simulink subsystem "controller_skeleton_FILTERED"  (R2023b)
settings: Solver=FixedStepDiscrete  StartTime=0.0  StopTime=10.0  RelTol=1e-3  EnableMultiTasking=on
values from neighbouring files (symbols this model uses):
  tvs =     [tvs_parameters.mat]
settings Model: Creator=Inver  LastModifiedBy=Inver
settings SolverCC: AutoInsertRateTranBlk=on
settings DataIOCC: SaveOutput=off  SaveTime=off
settings OptimizationCC: DefaultParameterBehavior=Inlined  InlineInvariantSignals=on  EnhancedBackFolding=on  PassReuseOutputArgsAs=Individual arguments  StateBitsets=on  DataBitsets=on  ZeroExternalMemoryAtStartup=off  ZeroInternalMemoryAtStartup=off  NoFixptDivByZeroProtection=on  LifeSpan=1  OptimizeBlockOrder=speed  DifferentSizesBufferReuse=on  EfficientTunableParamExpr=on
settings DebuggingCC: ParameterTunabilityLossMsg=error
settings HardwareCC: ProdBitPerPointer=32  ProdBitPerSizeT=32  ProdBitPerPtrDiffT=32  ProdLargestAtomicFloat=None  ProdIntDivRoundTo=Floor  ProdWordSize=32  ProdHWDeviceType=Generic->Custom
settings SFSimCC: MATLABDynamicMemAlloc=off
settings RTWCC: Description=Embedded Coder  SystemTargetFile=ert.tlc  TLCOptions=-p0  GenCodeOnly=on  TemplateMakefile=ert_default_tmf  GenerateReport=on  RTWVerbose=off  IncludeHyperlinkInReport=on  LaunchReport=on
settings CodeAppCC: ForceParamTrailComments=on  IgnoreCustomStorageClasses=off  OperatorAnnotations=on  SimulinkDataObjDesc=on  SFDataObjDesc=on  CustomSymbolStrGlobalVar=rt$N$M  CustomSymbolStrType=$N$M  CustomSymbolStrFcn=$N$M$F  CustomSymbolStrMacro=$N$M  InsertBlockDesc=on
settings ERTTargetCC: TargetLangStandard=C99 (ISO)  CodeReplacementLibrary=ISO_C  GenerateSampleERTMain=on  IncludeMdlTerminateFcn=off  SuppressErrorStatus=on  SupportAbsoluteTime=off  PurelyIntegerCode=on  SupportNonFinite=off  SupportComplex=off  InlinedParameterPlacement=NonHierarchical  RootIOFormat=Structure reference  ERTCustomFileTemplate=example_file_process.tlc

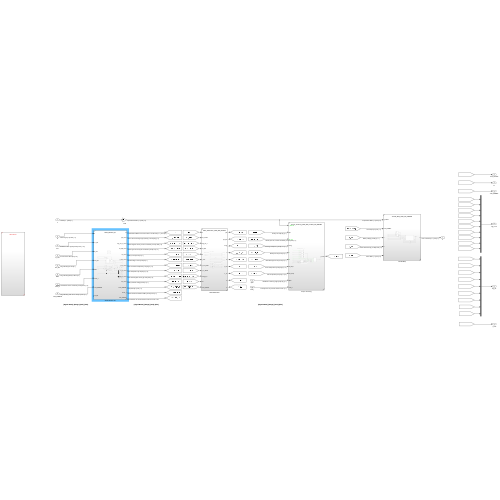
[thumbnail: Simulink's stored preview of the top-level diagram]
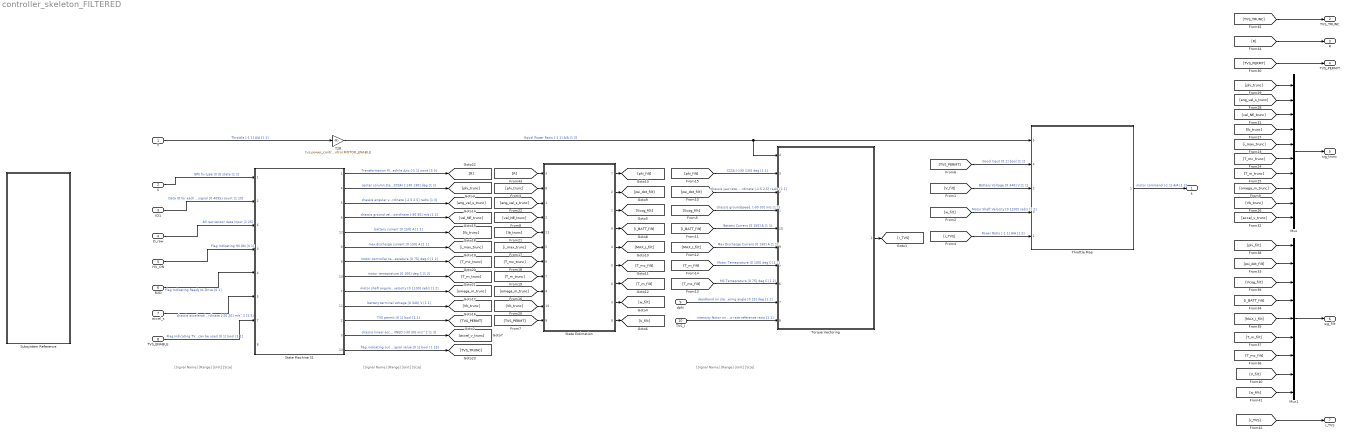
== system controller_skeleton_FILTERED ==
  note: [Signal Name] [Range] [Unit] [Size]
  note: [Signal Name] [Range] [Unit] [Size]
  note: [Signal Name] [Range] [Unit] [Size]
  T : Inport
  S : Inport  Port=2
  ID1 : Inport  Port=3
  D_raw : Inport  Port=4
  HV_ON : Inport  Port=5
  R2D : Inport  Port=6
  accel_s : Inport  Port=7
  TVS_ENABLE : Inport  Port=8
  dphi : Inport  Port=9
  TVS_I : Inport  Port=10
  Mux : Mux  Inputs=10
  Mux1 : Mux  Inputs=9
  State Estimation : Subsystem  ReferencedSubsystem=State_Estimation_2WD_NO_REGEN
      settings: PortSchema="{\"entries\":[{\"content\":{\"sides\":[{\"content\":{\"connectorIds\":[\"In3\",\"In8\",\"In1\",\"In2\",\"In11\",\"In5\",\"In6\",\"In7\",\"In4\",\"In10\",\"In9\"]},\"type\":\"ConnectorPlacement.EquallySpacedRectSide\",\"uuid\":\"a788c4af-c868-4742-81ae-137d8550b7dd\"},{\"content\":{\"connectorIds\":[\"Out7\",\"Out2\",\"Out1\",\"Out9\",\"Out4\",\"Out5\",\"Out6\",\"Out3\",\"Out8\"],\"side\":\"RIGHT\"},\"type\":\"ConnectorPlacement.EquallySpacedRectSide\",\"uuid\":\"40c1d3ed-7f96-4f50-8201-1fa73cbd293c\"},{\"content\":{\"side\":\"TOP\"},\"type\":\"ConnectorPlacement.EquallySpacedRectSide\",\"uuid\":\"412486a9-9897-40de-926c-efa6067c47b5\"}]},\"type\":\"ConnectorPlacement.EquallySpacedConnector\",\"uuid\":\"e2349428-ea4b-4d6c-9a0f-70e14711b204\"}],\"packageUris\":[\"http://schema.mathworks.com/mf0/Connector/R2020b\"],\"version\":\"1.0\"}"
  State Machine S1 : Subsystem  ReferencedSubsystem=State_Machine_S1
      settings: PortSchema="{\"entries\":[{\"content\":{\"sides\":[{\"content\":{\"connectorIds\":[\"In1\",\"In2\",\"In6\",\"In3\",\"In4\",\"In5\",\"In7\",\"In8\"]},\"type\":\"ConnectorPlacement.EquallySpacedRectSide\",\"uuid\":\"3ad5cc8f-5c24-495b-b7bf-c12b21ca6743\"},{\"content\":{\"connectorIds\":[\"Out1\",\"Out4\",\"Out5\",\"Out6\",\"Out12\",\"Out8\",\"Out9\",\"Out10\",\"Out7\",\"Out11\",\"Out2\",\"Out3\",\"Out13\"],\"side\":\"RIGHT\"},\"type\":\"ConnectorPlacement.EquallySpacedRectSide\",\"uuid\":\"199951c7-79be-4b7a-80a1-2c2fec8c516f\"},{\"content\":{\"side\":\"TOP\"},\"type\":\"ConnectorPlacement.EquallySpacedRectSide\",\"uuid\":\"296cd14f-6cd9-481e-92b9-c36b65280b3a\"}]},\"type\":\"ConnectorPlacement.EquallySpacedConnector\",\"uuid\":\"592bd7cc-8272-4bf2-9b34-0f5ee02d28bc\"}],\"packageUris\":[\"http://schema.mathworks.com/mf0/Connector/R2020b\"],\"version\":\"1.0\"}"
  Subsystem Reference : Subsystem  ReferencedSubsystem=<file name>
  T2R : Gain  Gain=tvs.power_control.ABS_MAX_POWER_RATIO.*tvs.power_control.MOTOR_ENABLE  OutDataTypeStr=double
  Throttle Map : Subsystem  ReferencedSubsystem=Throttle_Map_2WD_NO_REGEN
      settings: PortSchema="{\"entries\":[{\"content\":{\"sides\":[{\"content\":{\"connectorIds\":[\"In5\",\"In4\",\"In2\",\"In3\",\"In1\"]},\"type\":\"ConnectorPlacement.EquallySpacedRectSide\",\"uuid\":\"0a2325a3-9d51-4087-b02d-3e382446227a\"},{\"content\":{\"connectorIds\":[\"Out1\"],\"side\":\"RIGHT\"},\"type\":\"ConnectorPlacement.EquallySpacedRectSide\",\"uuid\":\"1dae26bb-0e0b-4c8e-9d40-43caeaa44005\"},{\"content\":{\"side\":\"TOP\"},\"type\":\"ConnectorPlacement.EquallySpacedRectSide\",\"uuid\":\"12710057-5a58-45a8-acf5-4b6ffc7139ef\"}]},\"type\":\"ConnectorPlacement.EquallySpacedConnector\",\"uuid\":\"fad868a8-f7f5-4d78-95c0-434c459d05fc\"}],\"packageUris\":[\"http://schema.mathworks.com/mf0/Connector/R2020b\"],\"version\":\"1.0\"}"
  Torque Vectoring : Subsystem  ReferencedSubsystem=Torque_Vectoring_2WD_NO_FILTER_NO_REGEN
      settings: PortSchema="{\"entries\":[{\"content\":{\"sides\":[{\"content\":{\"connectorIds\":[\"In4\",\"In3\",\"In2\",\"In1\",\"In10\",\"In9\",\"In5\",\"In6\",\"In7\",\"In8\"]},\"type\":\"ConnectorPlacement.EquallySpacedRectSide\",\"uuid\":\"e5337710-7afc-44d5-961b-efcd80b22325\"},{\"content\":{\"connectorIds\":[\"Out1\"],\"side\":\"RIGHT\"},\"type\":\"ConnectorPlacement.EquallySpacedRectSide\",\"uuid\":\"7e97e5bc-3983-40c2-bdf4-f229f862f80b\"},{\"content\":{\"side\":\"TOP\"},\"type\":\"ConnectorPlacement.EquallySpacedRectSide\",\"uuid\":\"1eebe57d-188b-4569-998a-307371d30e4f\"}]},\"type\":\"ConnectorPlacement.EquallySpacedConnector\",\"uuid\":\"25a81eaa-afe2-4445-a3db-4a69d15d4e62\"}],\"packageUris\":[\"http://schema.mathworks.com/mf0/Connector/R2020b\"],\"version\":\"1.0\"}"
  k : Outport
  TVS_TRUNC : Outport  Port=2
  R : Outport  Port=3
  TVS_PERMIT : Outport  Port=4
  sig_trunc : Outport  Port=5
  sig_filt : Outport  Port=6
  r_TVS : Outport  Port=7
  wires:
  T/1 -> T2R/1  "Throttle [-1 1] A/A [1 1]"
  [phi_trunc] -> State Estimation/8
  [ang_vel_s_trunc] -> State Estimation/1
  [vel_NE_trunc] -> State Estimation/2
  [omega_m_trunc] -> State Estimation/4
  [i_max_trunc] -> State Estimation/5
  [T_mc_trunc] -> State Estimation/6
  [T_m_trunc] -> State Estimation/7
  S/1 -> State Machine S1/1  "GPS fix type [0 3] state [1 1]"
  ID1/1 -> State Machine S1/2  "Data ID for each signal [0 4095] count [1 10]"
  Throttle Map/1 -> k/1  "motor command [-1 1] A/A [1 2]"
  [V_filt] -> Throttle Map/2  "Battery Voltage [0 340] V [1 1]"
  [w_filt] -> Throttle Map/3  "Motor Shaft Velocity [0 1200] rad/s [1 2]"
  dphi/1 -> Torque Vectoring/7  "deadband on steering angle [0 25] deg [1 1]"
  TVS_I/1 -> Torque Vectoring/8  "intensity factor on yaw rate reference ratio [1 1]"
  State Estimation/2 -> [psi_dot_filt]
  Torque Vectoring/1 -> [r_TVS]
  HV_ON/1 -> State Machine S1/3  "Flag Indicating HV ON [0 1]"
  R2D/1 -> State Machine S1/4  "Flag Indicating Ready to Drive [0 1]"
  accel_s/1 -> State Machine S1/5  "chassis acceleration sensor coordinate [-20 20] m/s^2 [1 3]"
  State Machine S1/1 -> [R]  "Transformation Matrix from Sensor Axis to Vechile Axis [-1 1] none [3 3]"
  [phi_filt] -> Torque Vectoring/3  "CCSA [-130 130] deg [1 1]"
  [T_m_filt] -> Torque Vectoring/5  "Motor Temeprature [0 100] deg C [1 2]"
  [T_mc_filt] -> Torque Vectoring/6  "MC Temeprature [0 75] deg C [1 2]"
  [MAX_I_filt] -> Torque Vectoring/9  "Max Discharge Current [0 150] A [1 1]"
  State Estimation/3 -> [w_filt]
  State Estimation/1 -> [Vcog_filt]
  [Vcog_filt] -> Torque Vectoring/1  "chassis groundspeed, [-30 30] m/s [1 1]"
  [Vb_trunc] -> State Estimation/10
  State Estimation/8 -> [V_filt]
  [Ib_trunc] -> State Estimation/11
  [I_BATT_filt] -> Torque Vectoring/10  "Battery Current [0 150] A [1 1]"
  [TVS_PERMT] -> Throttle Map/4  "Good Input [0 1] bool [1 1]"
  [r_TVS] -> Throttle Map/1  "Power Ratio [-1 1] A/A [1 2]"
  State Machine S1/3 -> [accel_v_trunc]  "chassis linear acceleration VNED [-30 30] m/s^2 [1 3]"
  T2R/1 -> Torque Vectoring/4, Throttle Map/5  "Equal Power Ratio [-1 1] A/A [1 2]"
  [psi_dot_filt] -> Torque Vectoring/2  "chassis yaw rate, vehicle coordinate [-2.5 2.5] rad/s [1 1]"
  State Estimation/9 -> [I_BATT_filt]
  State Estimation/4 -> [MAX_I_filt]
  State Estimation/5 -> [T_mc_filt]
  State Estimation/6 -> [T_m_filt]
  State Estimation/7 -> [phi_filt]
  D_raw/1 -> State Machine S1/6  "All raw sensor data input [1 25]"
  State Machine S1/2 -> [TVS_PERMT]  "TVS permit [0 1] bool [1 1]"
  TVS_ENABLE/1 -> State Machine S1/7  "Flag Indicating TVS can be used [0 1] bool [1 1]"
  State Machine S1/4 -> [phi_trunc]  "center column steering angle (CCSA) [-130 130] deg [1 1]"
  State Machine S1/5 -> [ang_vel_s_trunc]  "chassis angular velocity, sensor coordinate [-2.5 2.5] rad/s [1 3]"
  State Machine S1/6 -> [vel_NE_trunc]  "chassis ground velocity, NE coordinate [-30 30] m/s [1 2]"
  State Machine S1/11 -> [Vb_trunc]  "battery terminal voltage [0 340] V [1 1]"
  State Machine S1/10 -> [T_m_trunc]  "motor temeprature [0 100] deg C [1 2]"
  State Machine S1/9 -> [T_mc_trunc]  "motor controller temeprature [0 75] deg C [1 2]"
  State Machine S1/8 -> [i_max_trunc]  "max discharge current [0 150] A [1 1]"
  State Machine S1/12 -> [Ib_trunc]  "battery current [0 150] A [1 1]"
  State Machine S1/7 -> [omega_m_trunc]  "motor shaft angular velocity [0 1100] rad/s [1 2]"
  [TVS_PERMT] -> State Estimation/9
  [R] -> State Estimation/3
  [R] -> R/1
  [omega_m_trunc] -> Mux/8
  [phi_trunc] -> Mux/1
  [ang_vel_s_trunc] -> Mux/2
  [vel_NE_trunc] -> Mux/3
  [Ib_trunc] -> Mux/4
  [i_max_trunc] -> Mux/5
  [T_mc_trunc] -> Mux/6
  [T_m_trunc] -> Mux/7
  [Vb_trunc] -> Mux/9
  [accel_v_trunc] -> Mux/10
  [w_filt] -> Mux1/9
  [V_filt] -> Mux1/8
  [T_mc_filt] -> Mux1/7
  [T_m_filt] -> Mux1/6
  [MAX_I_filt] -> Mux1/5
  [I_BATT_filt] -> Mux1/4
  [Vcog_filt] -> Mux1/3
  [psi_dot_filt] -> Mux1/2
  [phi_filt] -> Mux1/1
  Mux/1 -> sig_trunc/1
  Mux1/1 -> sig_filt/1
  [TVS_PERMT] -> TVS_PERMIT/1
  [r_TVS] -> r_TVS/1
  State Machine S1/13 -> [TVS_TRUNC]  "flag indicating out of bounds signal value [0 1] bool [1 25]"
  [TVS_TRUNC] -> TVS_TRUNC/1

== system controller_skeleton_FILTERED/Subsystem Reference ==
